simulink library "app"  (Simulink 8.2)
settings: Solver=ode45  SolverMode=SingleTasking  StartTime=0.0  StopTime=10.0  RelTol=1e-3
PostLoadFcn:
  | , if any(exist('dsrtsu_mdlpostloadfcn', 'file') == [2, 3, 6]), try dsrtsu_mdlpostloadfcn('Execute', bdroot); catch fprintf('Error in PostLoadFcn (dsrtsu_mdlpostloadfcn) for model "%s":\n %s\n', bdroot, lasterr); end, end,
undefined symbols (not defined in the file or in its folder): C_TICK_TIME_S
libraries: simulink x2, acc x1, ada x1, aeb x1, ahlb x1, ddm x1, dfr x1, dgi x1, dhp x1, dinr x1, dip x1, dyn x1
settings Model: DSRTSU_INTERNAL_RTI_VER=450  DSRTSU_INTERNAL_RTI_TYPE=rti1401  RTICANMMDATA=struct('GeneralSetupData',struct('modelroot','C:\ADAS\trunk\ADAS_Softwares\HTDragon\software\sw_development\arch\app','generalsettings',struct('filesettings',struct('destfolder',struct('Name','RTICANMM_FILES','Check',1),'buildfolder',struct('Name','.','Check',1),'AbsDestfolder',struct('Name','C:\ADAS\trunk\ADAS_Softwares\HTDragon\software\sw_development\arch\app\RTICANMM_FILES'),'AbsBuildfolder',struct('Name','C:\ADAS\trunk\ADAS_Softwares\HTDragon\software\sw_development\arch\app'))),'options',struct('addpaths',1,'rmpaths',1,'addtrcexclusion',logical(1),'cannavigator',struct('checkmonitoring',0),'show_usrtrc',0,'use_usrtrc',0),'advanced',struct('options',[1 1 1 1 1 1 1 1 1 1 1 1 1 1 1 1 1 1 1 1 1 1 1 1 1 1 1 1 1 1 1 1 1 1 1 1 1 1 1 1 1 1 1 1 1 1 1 1 1 1 1 1 1 1 1 1 1 1 1 1 1 1 1 1 1 1 1 1 1 1 1 1 1 1 1 1 1 1 1 1 1 1 1 1 1 1 1 1 1 1 1 1 1 1 1 1 1 1 1 1]),'MPSetup',{{}},'modelname','app','block','app'))  DSRTSU_INTERNAL_RTIFPGA=40  Creator=jc19  LastModifiedBy=13192

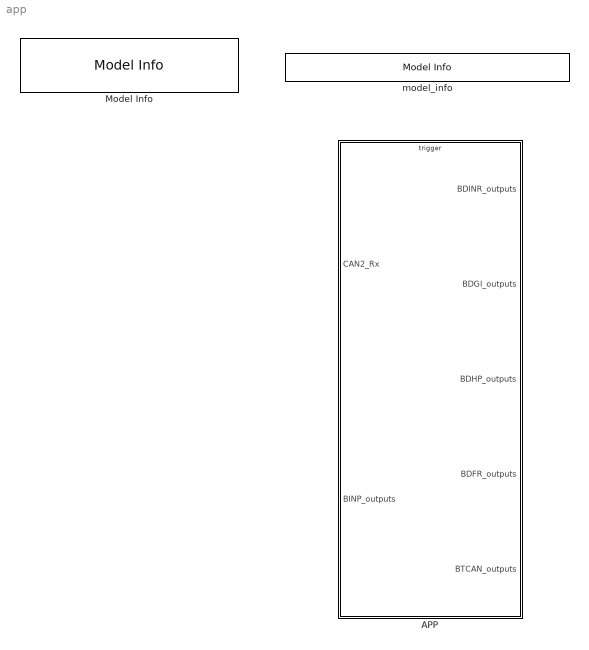
== system app ==
  APP : Subsystem
      settings: RTWSystemCode=Nonreusable function  RTWFcnNameOpts=Use subsystem name  RTWFileNameOpts=Use subsystem name
  Model Info : simulink/Model-Wide Utilities/Model Info  InitialBlockCM=None  BlockCM=None  Frame=on  DisplayStringWithTags=|  HorizontalTextAlignment=Left  LeftAlignmentValue=0.02  SourceBlockDiagram=app  TagMaxNumber=20
      | Model Version        : %<ModelVersion>
      | Creator                   : %<Creator>
      | Last Modified by    : %<LastModifiedBy>
  model_info : simulink/Model-Wide Utilities/Model Info  InitialBlockCM=None  BlockCM=None  Frame=on  DisplayStringWithTags=$Id: app.mdl 1622 2017-09-21 01:44:11Z bcluan $  HorizontalTextAlignment=Center  LeftAlignmentValue=0.5  SourceBlockDiagram=app  TagMaxNumber=20

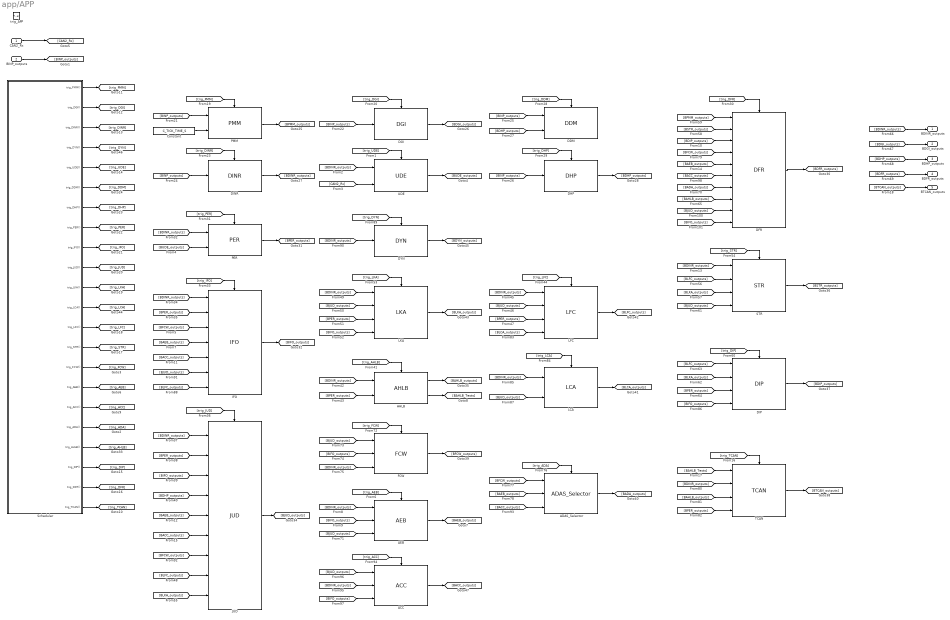
== system app/APP ==
  CAN2_Rx : Inport
  BINP_outputs : Inport  Port=2  OutDataTypeStr=Bus: BINP_outputs
      settings: LatchInputForFeedbackSignals=on
  trig_APP : TriggerPort  TriggerType=function-call
  ACC : acc/ACC
  ADAS_Selector : ada/ADAS_Selector
  AEB : aeb/AEB
  AHLB : ahlb/AHLB
  Constant : Constant  Value=C_TICK_TIME_S
  DDM : ddm/DDM
  DFR : dfr/DFR
  DGI : dgi/DGI
  DHP : dhp/DHP
  DINR : dinr/DINR
  DIP : dip/DIP
  DYN : dyn/DYN
  FCW : fcw/FCW
  IFO : ifo/IFO
  JUD : jud/JUD
  LCA : lca/LCA
  LFC : lfc/LFC
  LKA : lka/LKA
  PER : per/PER
  PMM : pmm/PMM
  STR : str/STR
  Scheduler : Stateflow chart  TreatAsAtomicUnit=on
  TCAN : tcan/TCAN
  UDE : ude/UDE
  BDINR_outputs : Outport  OutDataTypeStr=Bus: BDINR_outputs
  BDGI_outputs : Outport  Port=2  OutDataTypeStr=Bus: BDGI_outputs
  BDHP_outputs : Outport  Port=3  OutDataTypeStr=Bus: BDHP_outputs
  BDFR_outputs : Outport  Port=4  OutDataTypeStr=Bus: BDFR_outputs
  BTCAN_outputs : Outport  Port=5
  wires:
  [BIFO_outputs] -> DFR/10
  [CAN2_Rx] -> UDE/2
  BINP_outputs/1 -> [BINP_outputs]
  Scheduler/16(trig_AEB()) -> [trig_AEB]
  [trig_AEB] -> AEB/Trigger
  [BDINR_outputs] -> AEB/1
  [BIFO_outputs] -> AEB/2
  AEB/1 -> [BAEB_outputs]
  Scheduler/17(trig_ACC()) -> [trig_ACC]
  Scheduler/1(trig_PMM()) -> [trig_PMM]
  Scheduler/2(trig_DGI()) -> [trig_DGI]
  Scheduler/3(trig_DINR()) -> [trig_DINR]
  Scheduler/5(trig_UDE()) -> [trig_UDE]
  Scheduler/20(trig_DIP()) -> [trig_DIP]
  Scheduler/21(trig_DFR()) -> [trig_DFR]
  Scheduler/14(trig_STR()) -> [trig_STR]
  Scheduler/13(trig_LFC()) -> [trig_LFC]
  Scheduler/11(trig_LKA()) -> [trig_LKA]
  Scheduler/10(trig_JUD()) -> [trig_JUD]
  Scheduler/9(trig_IFO()) -> [trig_IFO]
  Scheduler/8(trig_PER()) -> [trig_PER]
  Scheduler/7(trig_DHP()) -> [trig_DHP]
  Scheduler/6(trig_DDM()) -> [trig_DDM]
  [trig_PMM] -> PMM/Trigger
  [BINP_outputs] -> PMM/1
  Constant/1 -> PMM/2
  PMM/1 -> [BPMM_outputs]
  [trig_DGI] -> DGI/Trigger
  [BINP_outputs] -> DGI/1
  DGI/1 -> [BDGI_outputs]
  [trig_DINR] -> DINR/Trigger
  [BINP_outputs] -> DINR/1
  DINR/1 -> [BDINR_outputs]
  [BINP_outputs] -> DDM/1
  [BINP_outputs] -> DHP/1
  [BDHP_outputs] -> DDM/2
  DHP/1 -> [BDHP_outputs]
  [trig_DDM] -> DDM/Trigger
  [trig_DHP] -> DHP/Trigger
  [trig_DFR] -> DFR/Trigger
  DFR/1 -> [BDFR_outputs]
  STR/1 -> [BSTR_outputs]
  [BPMM_outputs] -> DFR/1
  [trig_DIP] -> DIP/Trigger
  [BLFC_outputs] -> DIP/1
  DIP/1 -> [BDIP_outputs]
  [BDINR_outputs] -> BDINR_outputs/1
  [BDGI_outputs] -> BDGI_outputs/1
  [BDHP_outputs] -> BDHP_outputs/1
  [BDFR_outputs] -> BDFR_outputs/1
  [BDINR_outputs] -> STR/1
  [trig_PER] -> PER/Trigger
  [BDINR_outputs] -> PER/1
  PER/1 -> [BPER_outputs]
  [trig_IFO] -> IFO/Trigger
  [BDINR_outputs] -> IFO/1
  [BPER_outputs] -> IFO/2
  IFO/1 -> [BIFO_outputs]
  Scheduler/19(trig_AHLB()) -> [trig_AHLB]
  [trig_JUD] -> JUD/Trigger
  JUD/1 -> [BJUD_outputs]
  [BDINR_outputs] -> JUD/1
  [BPER_outputs] -> JUD/2
  [BIFO_outputs] -> JUD/3
  [BDHP_outputs] -> JUD/4
  [trig_AHLB] -> AHLB/Trigger
  AHLB/1 -> [BAHLB_outputs]
  [BDINR_outputs] -> AHLB/1
  [BPER_outputs] -> AHLB/2
  [trig_LFC] -> LFC/Trigger
  [BDINR_outputs] -> LFC/1
  [BJUD_outputs] -> LFC/2
  [BPER_outputs] -> LFC/3
  LFC/1 -> [BLFC_outputs]
  LKA/1 -> [BLKA_outputs]
  [BDINR_outputs] -> LKA/1
  [BJUD_outputs] -> LKA/2
  [BPER_outputs] -> LKA/3
  [BIFO_outputs] -> LKA/4
  [trig_LKA] -> LKA/Trigger
  [trig_STR] -> STR/Trigger
  [BLFC_outputs] -> STR/2
  [BLKA_outputs] -> STR/3
  [BJUD_outputs] -> STR/4
  [BLKA_outputs] -> DIP/2
  [BPER_outputs] -> DIP/3
  [trig_UDE] -> UDE/Trigger
  UDE/1 -> [BUDE_outputs]
  [BDINR_outputs] -> UDE/1
  CAN2_Rx/1 -> [CAN2_Rx]
  [BUDE_outputs] -> PER/2
  [BFCW_outputs] -> IFO/3
  [BAEB_outputs] -> IFO/4
  [BACC_outputs] -> IFO/5
  [BAEB_outputs] -> JUD/5
  [BACC_outputs] -> JUD/6
  AHLB/2 -> [BAHLB_Tests]
  Scheduler/15(trig_FCW()) -> [trig_FCW]
  Scheduler/18(trig_ADA()) -> [trig_ADA]
  Scheduler/22(trig_TCAN()) -> [trig_TCAN]
  TCAN/1 -> [BTCAN_outputs]
  [trig_TCAN] -> TCAN/Trigger
  [BAHLB_Tests] -> TCAN/1
  [BTCAN_outputs] -> BTCAN_outputs/1
  [BJUD_outputs] -> AEB/3
  [trig_FCW] -> FCW/Trigger
  [BJUD_outputs] -> FCW/1
  [BIFO_outputs] -> FCW/2
  [BDINR_outputs] -> FCW/3
  FCW/1 -> [BFCW_outputs]
  [trig_ADA] -> ADAS_Selector/Trigger
  [BFCW_outputs] -> ADAS_Selector/1
  [BAEB_outputs] -> ADAS_Selector/2
  ADAS_Selector/1 -> [BADA_outputs]
  [BDINR_outputs] -> TCAN/2
  [BAHLB_outputs] -> TCAN/3
  [BPER_outputs] -> TCAN/4
  LCA/1 -> [BLCA_outputs]
  [BLCA_outputs] -> LFC/4
  [trig_LCA] -> LCA/Trigger
  [BDINR_outputs] -> LCA/1
  [BJUD_outputs] -> LCA/2
  Scheduler/12(trig_LCA()) -> [trig_LCA]
  [trig_DYN] -> DYN/Trigger
  [BDINR_outputs] -> DYN/1
  DYN/1 -> [BDYN_outputs]
  Scheduler/4(trig_DYN()) -> [trig_DYN]
  [BJUD_outputs] -> IFO/6
  [BFCW_outputs] -> JUD/7
  [BLFC_outputs] -> JUD/8
  [BLKA_outputs] -> JUD/9
  [BACC_outputs] -> ADAS_Selector/3
  [trig_ACC] -> ACC/Trigger
  [BDINR_outputs] -> ACC/2
  [BIFO_outputs] -> ACC/3
  [BJUD_outputs] -> ACC/1
  ACC/1 -> [BACC_outputs]
  [BIFO_outputs] -> DIP/4
  [BLFC_outputs] -> IFO/7
  [BAHLB_outputs] -> DFR/8
  [BACC_outputs] -> DFR/6
  [BADA_outputs] -> DFR/7
  [BFCW_outputs] -> DFR/4
  [BAEB_outputs] -> DFR/5
  [BDIP_outputs] -> DFR/3
  [BSTR_outputs] -> DFR/2
  [BJUD_outputs] -> DFR/9

== stateflow chart APP/Scheduler ==
  (default) -> (junction 25)
  (junction 25) -> (junction 26) : {
      | trig_PMM; ...
      | trig_DGI; ...
      | trig_DINR; ...
      | trig_DYN; ...
      | trig_UDE; ...
      | trig_DDM; ...
      | trig_DHP; ...
      | trig_PER; ...
      | trig_IFO; ...
      | trig_JUD; ...
      | trig_LKA; ...
      | trig_LCA; ...
      | trig_LFC; ...
      | trig_STR; ...
      | trig_FCW; ...
      | trig_AEB; ...
      | trig_ACC; ...
      | trig_ADA; ...
      | trig_AHLB; ...
      | trig_DIP; ...
      | trig_DFR; ...
      | trig_TCAN; ...
      | }
  events: trig_PMM output FUNCTION_CALL_EVENT; trig_DGI output FUNCTION_CALL_EVENT; trig_DINR output FUNCTION_CALL_EVENT; trig_DYN output FUNCTION_CALL_EVENT; trig_UDE output FUNCTION_CALL_EVENT; trig_DDM output FUNCTION_CALL_EVENT; trig_DHP output FUNCTION_CALL_EVENT; trig_PER output FUNCTION_CALL_EVENT; trig_IFO output FUNCTION_CALL_EVENT; trig_JUD output FUNCTION_CALL_EVENT; trig_LKA output FUNCTION_CALL_EVENT; trig_LCA output FUNCTION_CALL_EVENT; trig_LFC output FUNCTION_CALL_EVENT; trig_STR output FUNCTION_CALL_EVENT; trig_FCW output FUNCTION_CALL_EVENT; trig_AEB output FUNCTION_CALL_EVENT; trig_ACC output FUNCTION_CALL_EVENT; trig_ADA output FUNCTION_CALL_EVENT; trig_AHLB output FUNCTION_CALL_EVENT; trig_DIP output FUNCTION_CALL_EVENT; trig_DFR output FUNCTION_CALL_EVENT; trig_TCAN output FUNCTION_CALL_EVENT
